simulink model "ABC_LMS"  (R2017a)
settings: Solver=VariableStepAuto  StartTime=0.0  StopTime=100  FixedStep=0.01  RelTol=1e-3  EnableMultiTasking=on
libraries: simulink x1, dsparch4 x1
settings Model: Creator=Gao Yuanyuan  LastModifiedBy=12867
settings OptimizationCC: LifeSpan=inf
settings DebuggingCC: SFUnexpectedBacktrackingDiag=warning  SFNoUnconditionalDefaultTransitionDiag=warning  SFExecutionAtInitializationDiag=none
settings GRTTargetCC: TargetLangStandard=C89/C90 (ANSI)  GeneratePreprocessorConditionals=Disable all
settings ConfigComp: CovMetricSettings=dw  CovHtmlReporting=on  CovSaveCumulativeToWorkspaceVar=on  CovSaveSingleToWorkspaceVar=on  CovExternalEMLEnable=off

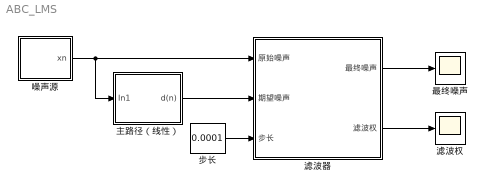
== system ABC_LMS ==
  主路径（线性） : Subsystem
  噪声源 : Subsystem
  "最终噪声 " : Scope
  步长 : Constant  Value=0.0001
  滤波器 : Subsystem
  滤波权 : Scope
  wires:
  滤波器/1(最终噪声) -> "最终噪声 "/1
  主路径（线性）/1(d(n)) -> 滤波器/2(期望噪声)
  步长/1 -> 滤波器/3(步长)
  噪声源/1(xn) -> 主路径（线性）/1(In1), 滤波器/1("原始噪声 ")
  滤波器/2(滤波权) -> 滤波权/1

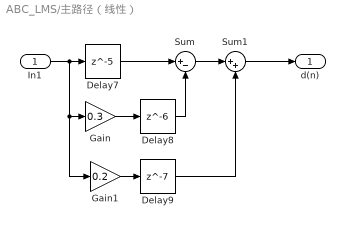
== system ABC_LMS/主路径（线性） ==
  In1 : Inport
  Delay7 : Delay  DelayLength=5  InitialCondition=0
  Delay8 : Delay  DelayLength=6  InitialCondition=0
  Delay9 : Delay  DelayLength=7  InitialCondition=0
  Gain : Gain  Gain=0.3
  Gain1 : Gain  Gain=0.2
  Sum : Sum  Inputs=|+-
  Sum1 : Sum  Inputs=|++
  d(n) : Outport
  wires:
  Gain/1 -> Delay8/1
  Sum/1 -> Sum1/1
  Gain1/1 -> Delay9/1
  In1/1 -> Delay7/1, Gain1/1, Gain/1
  Delay7/1 -> Sum/1
  Delay8/1 -> Sum/2
  Delay9/1 -> Sum1/2
  Sum1/1 -> d(n)/1

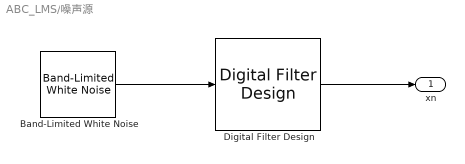
== system ABC_LMS/噪声源 ==
  Band-Limited White Noise : simulink/Sources/Band-Limited White Noise  Cov=[0.1]  Ts=0.0001  seed=[23341]
  Digital Filter Design : dsparch4/Digital Filter Design  mwdsp_browser_bugfix_var=off
  xn : Outport
  wires:
  Digital Filter Design/1 -> xn/1
  Band-Limited White Noise/1 -> Digital Filter Design/1

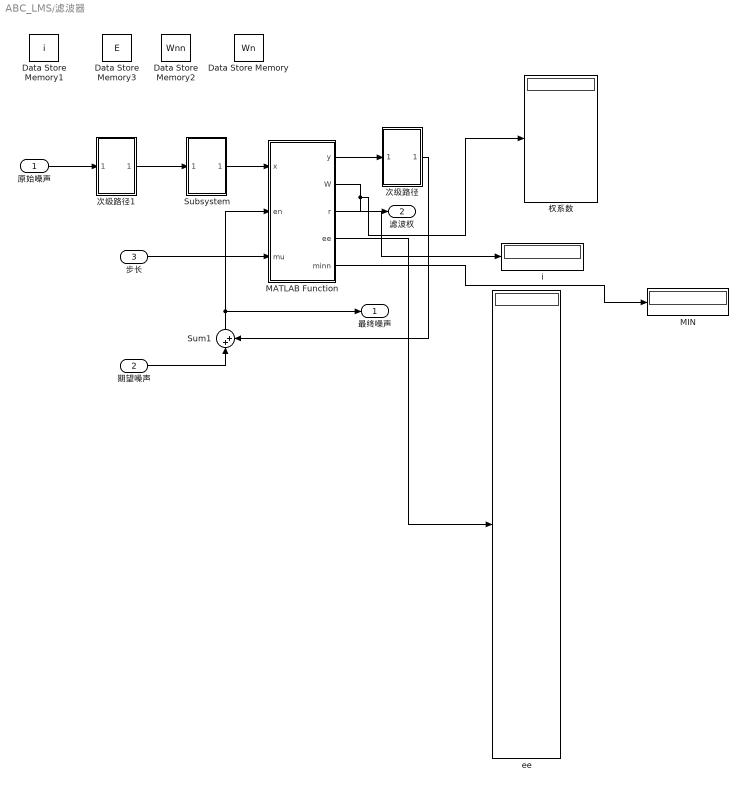
== system ABC_LMS/滤波器 ==
  "原始噪声 " : Inport
  期望噪声 : Inport  Port=2
  步长 : Inport  Port=3
  Data Store Memory : DataStoreMemory  DataStoreName=Wn  ReadBeforeWriteMsg=warning  WriteAfterWriteMsg=warning  WriteAfterReadMsg=warning  InitialValue=[0 0 0 0 0 0 0 0]  ShowAdditionalParam=off  OutDataTypeStr=double
  Data Store Memory1 : DataStoreMemory  DataStoreName=i  ReadBeforeWriteMsg=warning  WriteAfterWriteMsg=warning  WriteAfterReadMsg=warning  ShowAdditionalParam=off  OutDataTypeStr=double
  Data Store Memory2 : DataStoreMemory  DataStoreName=Wnn  ReadBeforeWriteMsg=warning  WriteAfterWriteMsg=warning  WriteAfterReadMsg=warning  InitialValue=[0 0 0 0 0 0 0 0;0 0 0 0 0 0 0 0;0 0 0 0 0 0 0 0;0 0 0 0 0 0 0 0;0 0 0 0 0 0 0 0;0 0 0 0 0 0 0 0;0 0 0 0 0 0 0 0;0 0 0 0 0 0 0 0;0 0 0 0 0 0 0 0;0 0 0 0 0 0 0 0;0 0 0 0 0 0 0 0;0 0 0 0 0 0 0 0;0 0 0 0 0 0 0 0;0 0 0 0 0 0 0 0;0 0 0 0 0 0 0 0;0 0 0 0 0 0 0 0;0 0 0 0 0 0 0 0;0 0 0 0 0 0 0 0;0 0 0 0 0 0 0 0;0 0 0 0 0 0 0 0;0 0 0 0 0 0 0 0;0 0 0 0 0 0 0 0;0 0 0 0 0 0 0 0;0 0 0 0 0 0 0 0;0 0 0 0 0 0 0 0;0 0 0 0 0 0 0 0;0 0 0 0 0 0 0 0;0 0 0 0 0 0 0 0;0 0 0 0 0 0 0 0;0 0 0 0 0 0 0 0;]  ShowAdditionalParam=off  OutDataTypeStr=double
  Data Store Memory3 : DataStoreMemory  DataStoreName=E  ReadBeforeWriteMsg=warning  WriteAfterWriteMsg=warning  WriteAfterReadMsg=warning  InitialValue=[0 0 0 0 0 0 0 0 0 0 0 0 0 0 0 0 0 0 0 0 0 0 0 0 0 0 0 0 0 0]  ShowAdditionalParam=off  OutDataTypeStr=double
  MATLAB Function : MATLAB Function  TreatAsAtomicUnit=on
  MIN : Display
  Subsystem : Subsystem
  Sum1 : Sum  Inputs=|++
  ee : Display
  i : Display
  权系数 : Display
  次级路径 : Subsystem
  次级路径1 : Subsystem
  最终噪声 : Outport
  滤波权 : Outport  Port=2
  wires:
  步长/1 -> MATLAB Function/3(mu)
  Sum1/1 -> MATLAB Function/2(en), 最终噪声/1
  期望噪声/1 -> Sum1/1
  Subsystem/1(Out1) -> MATLAB Function/1(x)
  MATLAB Function/1(y) -> 次级路径/1(In1)
  次级路径/1(Out1) -> Sum1/2
  "原始噪声 "/1 -> 次级路径1/1(In1)
  次级路径1/1(Out1) -> Subsystem/1(In1)
  MATLAB Function/3(r) -> i/1
  MATLAB Function/4(ee) -> ee/1
  MATLAB Function/2(W) -> 权系数/1, 滤波权/1
  MATLAB Function/5(minn) -> MIN/1

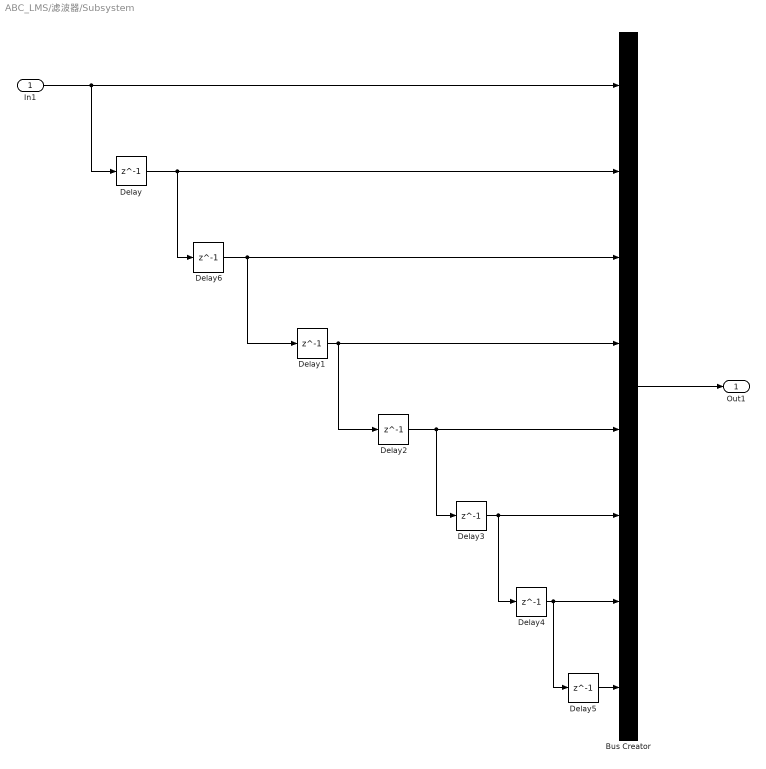
== system ABC_LMS/滤波器/Subsystem ==
  In1 : Inport
  Bus Creator : BusCreator  Inputs=8
  Delay{,1..6} (7 alike) : Delay  DelayLength=1  InitialCondition=0
  Out1 : Outport
  wires:
  Bus Creator/1 -> Out1/1
  Delay1/1 -> Delay2/1, Bus Creator/4
  Delay3/1 -> Bus Creator/6, Delay4/1
  Delay4/1 -> Delay5/1, Bus Creator/7
  Delay/1 -> Delay6/1, Bus Creator/2
  Delay6/1 -> Delay1/1, Bus Creator/3
  Delay5/1 -> Bus Creator/8
  In1/1 -> Delay/1, Bus Creator/1
  Delay2/1 -> Delay3/1, Bus Creator/5

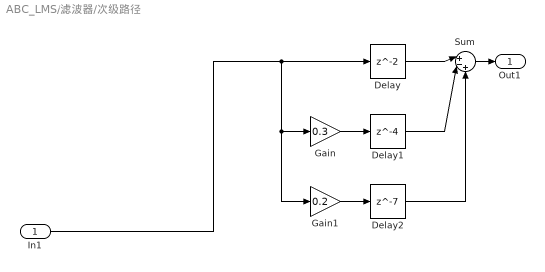
== system ABC_LMS/滤波器/次级路径 ==
  In1 : Inport
  Delay : Delay  InitialCondition=0
  Delay1 : Delay  DelayLength=4  InitialCondition=0
  Delay2 : Delay  DelayLength=7  InitialCondition=0
  Gain : Gain  Gain=0.3
  Gain1 : Gain  Gain=0.2
  Sum : Sum  Inputs=|+-+
  Out1 : Outport
  wires:
  Gain/1 -> Delay1/1
  Gain1/1 -> Delay2/1
  Delay2/1 -> Sum/3
  Delay1/1 -> Sum/2
  In1/1 -> Gain1/1, Gain/1, Delay/1
  Delay/1 -> Sum/1
  Sum/1 -> Out1/1

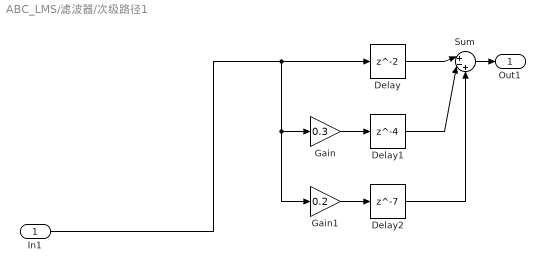
== system ABC_LMS/滤波器/次级路径1 ==
  In1 : Inport
  Delay : Delay  InitialCondition=0
  Delay1 : Delay  DelayLength=4  InitialCondition=0
  Delay2 : Delay  DelayLength=7  InitialCondition=0
  Gain : Gain  Gain=0.3
  Gain1 : Gain  Gain=0.2
  Sum : Sum  Inputs=|+-+
  Out1 : Outport
  wires:
  Gain/1 -> Delay1/1
  Gain1/1 -> Delay2/1
  Delay2/1 -> Sum/3
  Delay1/1 -> Sum/2
  In1/1 -> Gain1/1, Gain/1, Delay/1
  Delay/1 -> Sum/1
  Sum/1 -> Out1/1

== matlab function ABC_LMS/滤波器/MATLAB Function ==
  data: x input; y output; en input; mu input; Wn data_store_memory; W output; i data_store_memory; Wnn data_store_memory; E data_store_memory; r output; ee output; minn output
function [y,W,r,ee,minn] = fcn(x,en,mu)
global Wn;
global i;
global Wnn;%蜜源个数为30
global E;
 i=i+1;
 MIN=0;
if(i<=30)
    for j=1:8
       Wnn(i,j)=unifrnd(-0.5,0.5);
    end
    Wn=Wnn(i,:)';
    E(i)=en;
elseif(i==31) 
   MIN=min(abs(E(9:30)));
   for j=9:30
      if(abs(E(j))==MIN)
         Wn=Wnn(j-1,:)'; 
      end
   end
    Wn=Wn-mu*x*en;
else
     Wn=Wn-mu*x*en;
end
minn=MIN;

    y=Wn'*x;
    W=Wn;
    r=i;
    ee=E;
end
